simulink model "Indirect"  (R2015b)
settings: Solver=VariableStepAuto  StartTime=0.0  StopTime=7  RelTol=1e-3
values from neighbouring files (symbols this model uses):
  f = 50    [Indirect_init.m]
  L = XL/(2*2*pi*f)    (= 0.159154943092)    [Indirect_init.m]
  L_STATCOM = 44.56e-5    (= 0.0004456)    [Indirect_init.m]
  R_Statcom = 1e-1    (= 0.1)    [Indirect_init.m]
  Sbase = 1000e6/2    (= 500000000)    [Indirect_init.m]
  Ts = 10e-6    (= 1e-05)    [Indirect_init.m]
  Tsample = 200e-6    (= 0.0002)    [Indirect_init.m]
  Vr = 220e3    (= 220000)    [Indirect_init.m]
  Vs = 220e3    (= 220000)    [Indirect_init.m]
libraries: powerlib x27, powerlib_meascontrol x16, simulink x2
settings Model: Creator=Sourabh Suri  LastModifiedBy=Sourabh Suri

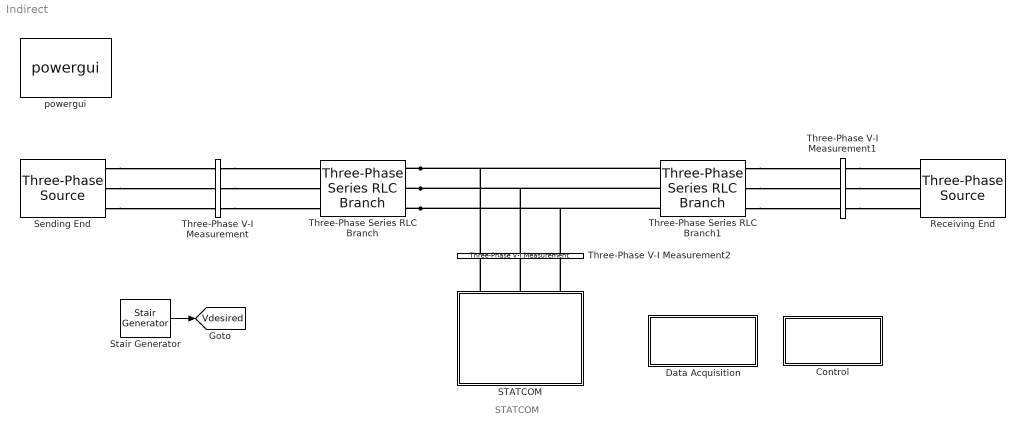
== system Indirect ==
  note: STATCOM
  Control : Subsystem
  Data Acquisition : Subsystem
  Receiving End : powerlib/Electrical Sources/Three-Phase Source  InternalConnection=Yg  VoltagePhases=off  Voltage=Vr  PhaseAngle=dr  Voltage_phases=[25e3 25e3 25e3]/sqrt(3)  PhaseAngles_phases=[0 -120 +120]  Frequency=f  NonIdealSource=off  SpecifyImpedance=off  Resistance=0.8929  Inductance=16.58e-3  ShortCircuitLevel=100e6  BaseVoltage=25e3  XRratio=7  BusType=swing  Pref=10e3  Qref=0  Prefabc=[10e3, 10e3, 10e3]  Qrefabc=[0, 0, 0]  Qmin=-inf  Qmax=inf
  STATCOM : Subsystem
  Sending End : powerlib/Electrical Sources/Three-Phase Source  InternalConnection=Yg  VoltagePhases=off  Voltage=Vs  PhaseAngle=ds  Voltage_phases=[25e3 25e3 25e3]/sqrt(3)  PhaseAngles_phases=[0 -120 +120]  Frequency=f  NonIdealSource=off  SpecifyImpedance=off  Resistance=0  Inductance=0  ShortCircuitLevel=100e6  BaseVoltage=0  XRratio=7  BusType=swing  Pref=10e3  Qref=0  Prefabc=[10e3, 10e3, 10e3]  Qrefabc=[0, 0, 0]  Qmin=-inf  Qmax=inf
  Stair Generator : powerlib_meascontrol/Pulse & Signal Generators/Stair Generator  t=[0:.5:.5*12]  e=[.07:.005:.13]  Ts=Ts
  Three-Phase Series RLC Branch : powerlib/Elements/Three-Phase Series RLC Branch  LConnTagsString=A|B|C  RConnTagsString=A|B|C  BranchType=L  Resistance=1  Inductance=L  Capacitance=1e-6  Measurements=None
  Three-Phase Series RLC Branch1 : powerlib/Elements/Three-Phase Series RLC Branch  LConnTagsString=A|B|C  RConnTagsString=A|B|C  BranchType=L  Resistance=1  Inductance=L  Capacitance=1e-6  Measurements=None
  Three-Phase V-I Measurement : powerlib/Measurements/Three-Phase V-I Measurement  VoltageMeasurement=phase-to-phase  SetLabelV=on  LabelV=Vsabc  Vpu=off  VpuLL=on  CurrentMeasurement=yes  SetLabelI=on  LabelI=Isabc  Ipu=on  Pbase=Sbase  Vbase=Vn  OutputType=Complex  PhasorSimulation=off  PSBequivalent=0
  Three-Phase V-I Measurement1 : powerlib/Measurements/Three-Phase V-I Measurement  VoltageMeasurement=phase-to-phase  SetLabelV=on  LabelV=Vrabc  Vpu=off  VpuLL=on  CurrentMeasurement=yes  SetLabelI=on  LabelI=Irabc  Ipu=on  Pbase=Sbase  Vbase=Vn  OutputType=Complex  PhasorSimulation=off  PSBequivalent=0
  Three-Phase V-I Measurement2 : powerlib/Measurements/Three-Phase V-I Measurement  VoltageMeasurement=phase-to-phase  SetLabelV=on  LabelV=Vmabc  Vpu=off  VpuLL=on  CurrentMeasurement=yes  SetLabelI=on  LabelI=Imabc  Ipu=on  Pbase=Sbase  Vbase=Vn  OutputType=Complex  PhasorSimulation=off  PSBequivalent=0
  powergui : powerlib/powergui  Priority=1  SimulationMode=Discrete  SolverType=Tustin/Backward Euler (TBE)  SampleTime=Ts  frequency=60  SPID=on  DisableSnubberDevices=on  DisableRonSwitches=on  DisableVfSwitches=on  SwTol=0  DisplayEquations=off  Interpol=off  ExternalGateDelay=off  methode=off  Ts=10  FunctionMessages=off  echomessages=off  HookPort=off  EnableUseOfTLC=off  x0status=blocks  frequencyindice=50  Pbase=100e6  ErrMax=1e-4  Iterations=50  UnitsV=kV  UnitsW=MW  buscounter=0  RestoreLinks=warning  ResistiveCurrentMeasurement=off  Frange=[0:2:500]  Ylog=off  Xlog=on  ShowGrid=off  save=off  variable=ZData  structure=0  ZoomFFT=off  StartTime=0.0  cycles=1  DisplayStyle=1  fundamental=60  FreqAxis=off  MaxFrequency=1000  frequencyindicesteady=1  RmsSteady=1  display=off
  tag scope: Vdesired=global
  wires:
  Stair Generator/1 -> [Vdesired]
  connections:
  Three-Phase Series RLC Branch/RConn1 -- Three-Phase Series RLC Branch1/RConn1 -- Three-Phase V-I Measurement2/RConn1
  Three-Phase Series RLC Branch/RConn2 -- Three-Phase Series RLC Branch1/RConn2 -- Three-Phase V-I Measurement2/RConn2
  Three-Phase Series RLC Branch/RConn3 -- Three-Phase Series RLC Branch1/RConn3 -- Three-Phase V-I Measurement2/RConn3
  Sending End/RConn1 -- Three-Phase V-I Measurement/LConn1
  Sending End/RConn2 -- Three-Phase V-I Measurement/LConn2
  Three-Phase V-I Measurement1/LConn2 -- Receiving End/RConn2
  Three-Phase Series RLC Branch1/LConn2 -- Three-Phase V-I Measurement1/RConn2
  Three-Phase V-I Measurement1/LConn1 -- Receiving End/RConn1
  Three-Phase Series RLC Branch1/LConn1 -- Three-Phase V-I Measurement1/RConn1
  Three-Phase V-I Measurement/RConn2 -- Three-Phase Series RLC Branch/LConn2
  Sending End/RConn3 -- Three-Phase V-I Measurement/LConn3
  Three-Phase V-I Measurement/RConn3 -- Three-Phase Series RLC Branch/LConn3
  Three-Phase Series RLC Branch1/LConn3 -- Three-Phase V-I Measurement1/RConn3
  Three-Phase V-I Measurement/RConn1 -- Three-Phase Series RLC Branch/LConn1
  Three-Phase V-I Measurement1/LConn3 -- Receiving End/RConn3
  STATCOM/LConn1 -- Three-Phase V-I Measurement2/LConn1
  STATCOM/LConn2 -- Three-Phase V-I Measurement2/LConn2
  STATCOM/LConn3 -- Three-Phase V-I Measurement2/LConn3

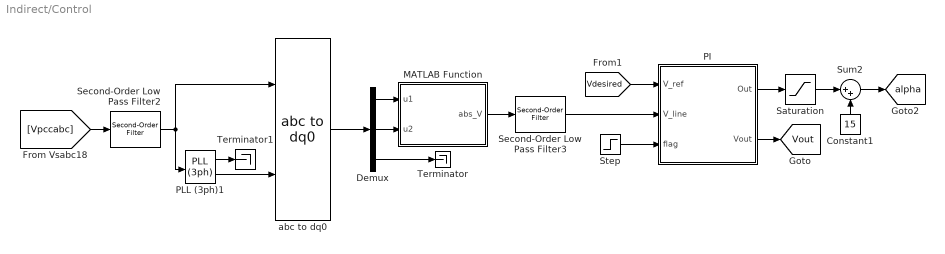
== system Indirect/Control ==
  Constant1 : Constant  Value=15
  Demux : Demux  Outputs=3
  MATLAB Function : MATLAB Function  TreatAsAtomicUnit=on
  PI : MATLAB Function  TreatAsAtomicUnit=on
  PLL (3ph)1 : powerlib_meascontrol/PLL/PLL (3ph)  Fmin=45  Par_Init=[3.7 50.1]  ParK=[60 1400 0]  TcD=1.6e-4  MaxRateChangeFreq=10  FilterCutOffFreq=25  Ts=Ts  AGC=on
  Saturation : Saturate  UpperLimit=45  LowerLimit=-15
  Second-Order Low Pass Filter2 : powerlib_meascontrol/Filters/Second-Order Filter  FilterType=Bandpass  Fo=50  Zeta=0.707  Ts=Ts  Initialize=off  Vac_Init="[0,  0,  60]"  Vdc_Init=0  PlotResponse=off  FreqRange=[0, 500, 1]
      settings: AttributesFormatString=f0: %<Fo>
  Second-Order Low Pass Filter3 : powerlib_meascontrol/Filters/Second-Order Filter  FilterType=Lowpass  Fo=25  Zeta=0.707  Ts=Ts  Initialize=off  Vac_Init="[0,  0,  60]"  Vdc_Init=0  PlotResponse=off  FreqRange=[0, 50, 1]
      settings: AttributesFormatString=f0: %<Fo>
  Step : Step  Time=1.01/f  SampleTime=0
  Sum2 : Sum  Inputs=|++  SaturateOnIntegerOverflow=on  InputSameDT=on  OutDataTypeStr=Inherit: Same as first input
  Terminator : Terminator
  Terminator1 : Terminator
  abc to dq0 : powerlib_meascontrol/Transformations/abc to dq0  Alignment=90 degrees behind phase A axis
  tag scope: Vout=global, alpha=global
  wires:
  [Vdesired] -> PI/1(V_ref)
  PI/1(Out) -> Saturation/1
  Saturation/1 -> Sum2/1
  Sum2/1 -> [alpha]
  Constant1/1 -> Sum2/2
  Step/1 -> PI/3(flag)
  PLL (3ph)1/2 -> abc to dq0/2
  [Vpccabc] -> Second-Order Low Pass Filter2/1
  abc to dq0/1 -> Demux/1
  Demux/1 -> MATLAB Function/1(u1)
  Demux/2 -> MATLAB Function/2(u2)
  Demux/3 -> Terminator/1
  Second-Order Low Pass Filter2/1 -> abc to dq0/1, PLL (3ph)1/1
  MATLAB Function/1(abs_V) -> Second-Order Low Pass Filter3/1
  Second-Order Low Pass Filter3/1 -> PI/2(V_line)
  PLL (3ph)1/1 -> Terminator1/1
  PI/2(Vout) -> [Vout]

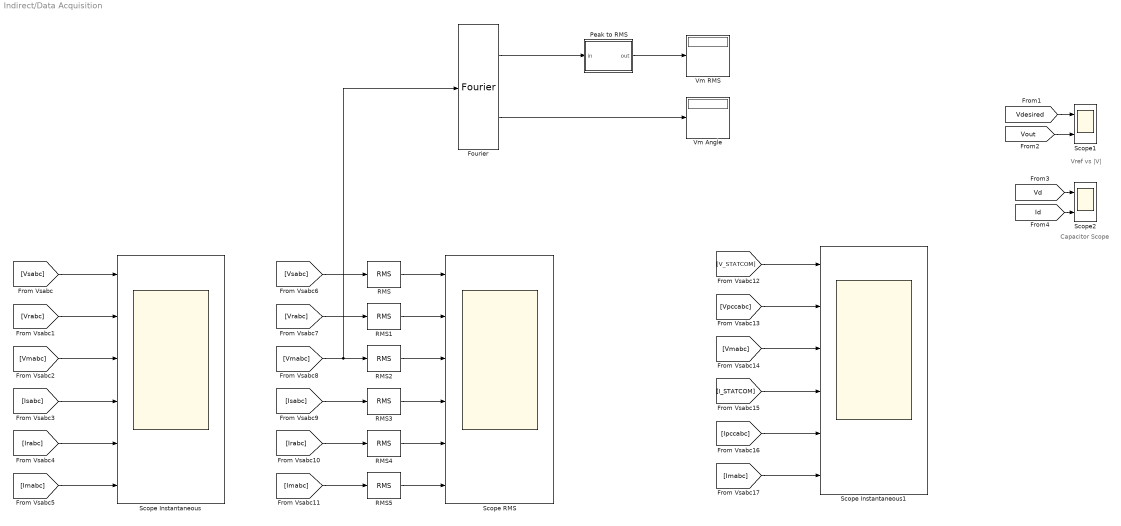
== system Indirect/Data Acquisition ==
  note: Vref vs |V|
  note: Capacitor Scope
  Fourier : powerlib_meascontrol/Measurements/Fourier  Freq=f  n=1  InInit=[0, 0]  Ts=0
  Peak to RMS : MATLAB Function  TreatAsAtomicUnit=on
  RMS{,1..5} (6 alike) : powerlib_meascontrol/Measurements/RMS  TrueRMS=off  Freq=f  RMSInit=0  Ts=0
  Scope Instantaneous : Scope  NumInputPorts=6
  Scope Instantaneous1 : Scope  NumInputPorts=6
  Scope RMS : Scope  NumInputPorts=6
  Scope1 : Scope  NumInputPorts=2
  Scope2 : Scope  NumInputPorts=2
  Vm Angle : Display
      settings: Decimation=3
  Vm RMS : Display
      settings: Decimation=3
  wires:
  [Vsabc] -> Scope Instantaneous/1
  [Vrabc] -> Scope Instantaneous/2
  [Irabc] -> Scope Instantaneous/5
  [Imabc] -> Scope Instantaneous/6
  [Vmabc] -> Scope Instantaneous/3
  [Isabc] -> Scope Instantaneous/4
  RMS/1 -> Scope RMS/1
  [Vrabc] -> RMS1/1
  RMS1/1 -> Scope RMS/2
  [Vmabc] -> Fourier/1, RMS2/1
  [Isabc] -> RMS3/1
  RMS3/1 -> Scope RMS/4
  [Irabc] -> RMS4/1
  RMS4/1 -> Scope RMS/5
  [Imabc] -> RMS5/1
  RMS5/1 -> Scope RMS/6
  RMS2/1 -> Scope RMS/3
  Fourier/2 -> Vm Angle/1
  [Vsabc] -> RMS/1
  Peak to RMS/1(out) -> Vm RMS/1
  Fourier/1 -> Peak to RMS/1(in)
  [Vdesired] -> Scope1/1
  [Vout] -> Scope1/2
  [Vd] -> Scope2/1
  [Id] -> Scope2/2
  [V_STATCOM] -> Scope Instantaneous1/1
  [Vpccabc] -> Scope Instantaneous1/2
  [Ipccabc] -> Scope Instantaneous1/5
  [Imabc] -> Scope Instantaneous1/6
  [Vmabc] -> Scope Instantaneous1/3
  [I_STATCOM] -> Scope Instantaneous1/4
  ? -> ?

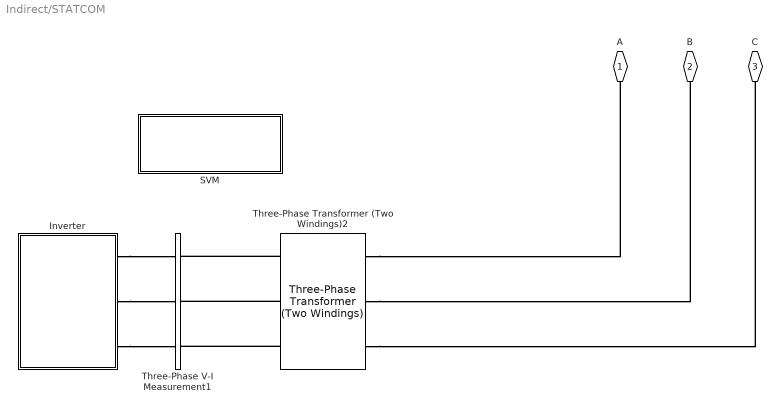
== system Indirect/STATCOM ==
  Inverter : Subsystem
  SVM : Subsystem
  Three-Phase Transformer (Two Windings)2 : powerlib/Elements/Three-Phase Transformer (Two Windings)  Winding1Connection=Y  Winding2Connection=Y  CoreType=Three-limb core (core-type)  SetSaturation=off  Hysteresis=off  DataFile='hysteresis'  SetInitialFlux=off  Measurements=None  UNITS=SI  NominalPower=[ Sbase*1000 , 50 ]  Winding1=[22e+04 1e-9 0 ]  Winding2=[22e+03 1e-9 0]  Rm=inf  Lm=inf  L0=0.5  Saturation=[0 0;4.3111 686.13;1796.3 869.1]  InitialFluxes=[457.42 -457.42 400.24]  MoreParameters=off  BreakLoop=off  DataType=on  TransfoNumber=1
  Three-Phase V-I Measurement1 : powerlib/Measurements/Three-Phase V-I Measurement  VoltageMeasurement=phase-to-phase  SetLabelV=on  LabelV=Vpccabc  Vpu=off  VpuLL=on  CurrentMeasurement=yes  SetLabelI=on  LabelI=Ipccabc  Ipu=on  Pbase=Sbase  Vbase=Vn  OutputType=Complex  PhasorSimulation=off  PSBequivalent=0
  A : PMIOPort  Port=1  Side=Left
  B : PMIOPort  Port=2  Side=Left
  C : PMIOPort  Port=3  Side=Left
  connections:
  Three-Phase Transformer (Two Windings)2/LConn1 -- A/RConn1
  Three-Phase Transformer (Two Windings)2/LConn2 -- B/RConn1
  Three-Phase Transformer (Two Windings)2/LConn3 -- C/RConn1
  Three-Phase Transformer (Two Windings)2/RConn1 -- Three-Phase V-I Measurement1/RConn1
  Three-Phase Transformer (Two Windings)2/RConn2 -- Three-Phase V-I Measurement1/RConn2
  Three-Phase Transformer (Two Windings)2/RConn3 -- Three-Phase V-I Measurement1/RConn3
  Inverter/LConn1 -- Three-Phase V-I Measurement1/LConn1
  Inverter/LConn2 -- Three-Phase V-I Measurement1/LConn2
  Inverter/LConn3 -- Three-Phase V-I Measurement1/LConn3

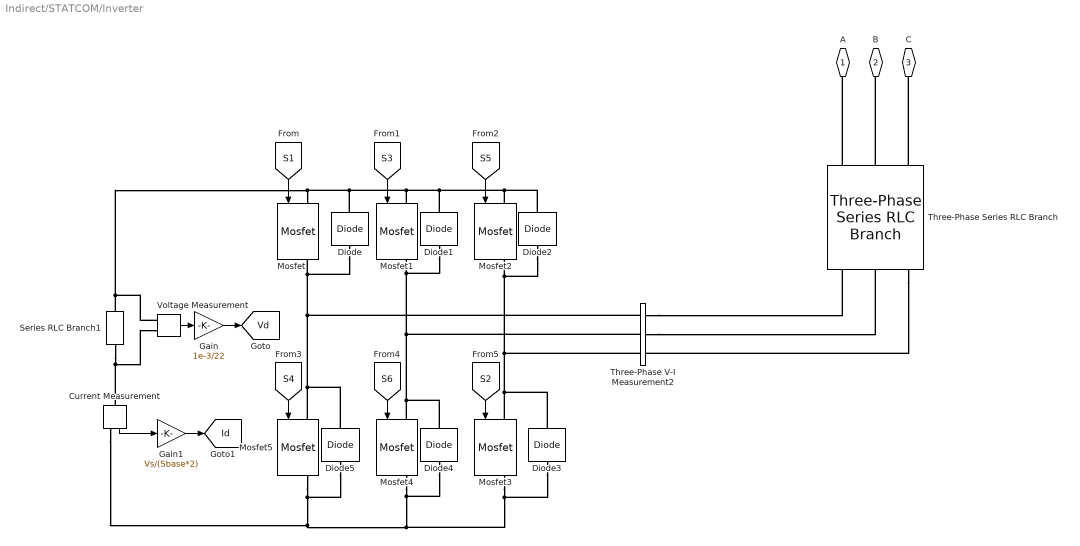
== system Indirect/STATCOM/Inverter ==
  Current Measurement : powerlib/Measurements/Current Measurement  PhasorSimulation=off  OutputType=Complex  PSBequivalent=0
  Diode{,1..5} (6 alike) : powerlib/Power Electronics/Diode  Ron=0.001  Lon=0  Vf=0.8  IC=0  UseSnubber=off  Rs=inf  Cs=250e-9  Measurements=off
  Gain : Gain  Gain=1e-3/22
  Gain1 : Gain  Gain=Vs/(Sbase*2)
  Mosfet{,1..5} (6 alike) : powerlib/Power Electronics/Mosfet  Ron=0.1  Lon=0  Rd=0.01  Vfd=0  IC=0  Rs=1e5  Cs=inf  Measurements=on
  Series RLC Branch1 : powerlib/Elements/Series RLC Branch  LConnTagsString=__new0  RConnTagsString=__new0  BranchType=C  Resistance=100  Inductance=1e-15  SetiL0=off  InitialCurrent=0  Capacitance=20e-4  Setx0=on  InitialVoltage=22e3/.45  Measurements=None
  Three-Phase Series RLC Branch : powerlib/Elements/Three-Phase Series RLC Branch  LConnTagsString=A|B|C  RConnTagsString=A|B|C  BranchType=RL  Resistance=R_Statcom  Inductance=L_STATCOM  Capacitance=1e-6  Measurements=None
  Three-Phase V-I Measurement2 : powerlib/Measurements/Three-Phase V-I Measurement  VoltageMeasurement=phase-to-phase  SetLabelV=on  LabelV=V_STATCOM  Vpu=off  VpuLL=on  CurrentMeasurement=yes  SetLabelI=on  LabelI=I_STATCOM  Ipu=on  Pbase=Sbase  Vbase=Vn  OutputType=Complex  PhasorSimulation=off  PSBequivalent=0
  Voltage Measurement : powerlib/Measurements/Voltage Measurement  PhasorSimulation=off  OutputType=Complex  PSBequivalent=0
  A : PMIOPort  Port=1  Side=Left
  B : PMIOPort  Port=2  Side=Left
  C : PMIOPort  Port=3  Side=Left
  tag scope: Id=global, Vd=global
  wires:
  [S2] -> Mosfet3/1
  [S4] -> Mosfet5/1
  [S1] -> Mosfet/1
  [S5] -> Mosfet2/1
  [S3] -> Mosfet1/1
  [S6] -> Mosfet4/1
  Voltage Measurement/1 -> Gain/1
  Gain/1 -> [Vd]
  Gain1/1 -> [Id]
  Current Measurement/1 -> Gain1/1
  connections:
  Series RLC Branch1/RConn1 -- Current Measurement/LConn1 -- Voltage Measurement/LConn2
  Voltage Measurement/LConn1 -- Series RLC Branch1/LConn1 -- Mosfet/LConn1 -- Diode2/RConn1 -- Mosfet2/LConn1 -- Diode1/RConn1 -- Mosfet1/LConn1 -- Diode/RConn1
  Mosfet/RConn1 -- Three-Phase V-I Measurement2/LConn1 -- Diode5/RConn1 -- Mosfet5/LConn1 -- Diode/LConn1
  Mosfet1/RConn1 -- Three-Phase V-I Measurement2/LConn2 -- Diode4/RConn1 -- Mosfet4/LConn1 -- Diode1/LConn1
  Mosfet2/RConn1 -- Three-Phase V-I Measurement2/LConn3 -- Diode3/RConn1 -- Mosfet3/LConn1 -- Diode2/LConn1
  Three-Phase Series RLC Branch/LConn2 -- B/RConn1
  Three-Phase Series RLC Branch/LConn3 -- C/RConn1
  Three-Phase Series RLC Branch/LConn1 -- A/RConn1
  Three-Phase V-I Measurement2/RConn1 -- Three-Phase Series RLC Branch/RConn1
  Three-Phase V-I Measurement2/RConn2 -- Three-Phase Series RLC Branch/RConn2
  Three-Phase Series RLC Branch/RConn3 -- Three-Phase V-I Measurement2/RConn3
  Diode3/LConn1 -- Current Measurement/RConn1 -- Diode5/LConn1 -- Mosfet5/RConn1 -- Diode4/LConn1 -- Mosfet4/RConn1 -- Mosfet3/RConn1

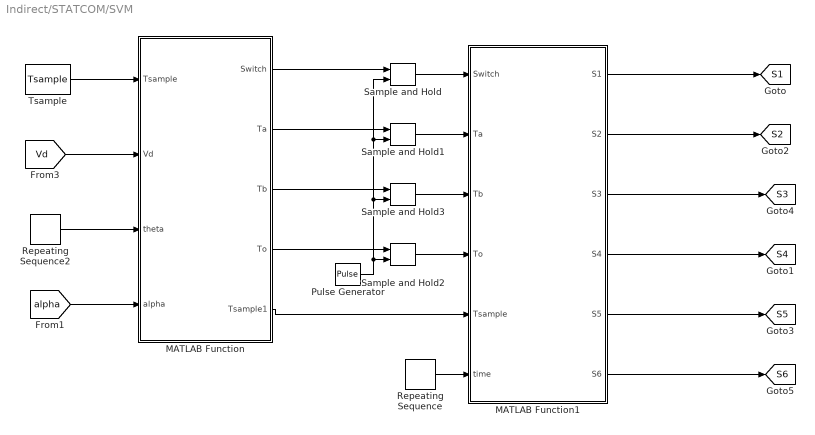
== system Indirect/STATCOM/SVM ==
  MATLAB Function : MATLAB Function  TreatAsAtomicUnit=on
  MATLAB Function1 : MATLAB Function  TreatAsAtomicUnit=on
  Pulse Generator : DiscretePulseGenerator  PulseType=Time based  Period=Tsample  PulseWidth=.1
  Repeating Sequence : simulink/Sources/Repeating Sequence  rep_seq_t=[0 Tsample ]  rep_seq_y=[0 Tsample]
  Repeating Sequence2 : simulink/Sources/Repeating Sequence  rep_seq_t=[0 1/f ]  rep_seq_y=[0 (2*pi)]
  Sample and Hold{,1..3} (4 alike) : powerlib_meascontrol/Additional Components/Sample and Hold  ic=0  Ts=Tsample
  Tsample : Constant  Value=Tsample
  tag scope: S1=global, S2=global, S3=global, S4=global, S5=global, S6=global
  wires:
  MATLAB Function/1(Switch) -> Sample and Hold/1
  Sample and Hold/1 -> MATLAB Function1/1(Switch)
  MATLAB Function/3(Tb) -> Sample and Hold3/1
  MATLAB Function1/1(S1) -> [S1]
  MATLAB Function1/5(S5) -> [S5]
  MATLAB Function1/3(S3) -> [S3]
  MATLAB Function1/4(S4) -> [S4]
  MATLAB Function1/2(S2) -> [S2]
  Sample and Hold1/1 -> MATLAB Function1/2(Ta)
  MATLAB Function/2(Ta) -> Sample and Hold1/1
  Sample and Hold2/1 -> MATLAB Function1/4(To)
  MATLAB Function/4(To) -> Sample and Hold2/1
  Pulse Generator/1 -> Sample and Hold/2, Sample and Hold1/2, Sample and Hold3/2, Sample and Hold2/2
  MATLAB Function1/6(S6) -> [S6]
  Tsample/1 -> MATLAB Function/1(Tsample)
  Repeating Sequence/1 -> MATLAB Function1/6(time)
  MATLAB Function/5(Tsample1) -> MATLAB Function1/5(Tsample)
  [Vd] -> MATLAB Function/2(Vd)
  Sample and Hold3/1 -> MATLAB Function1/3(Tb)
  Repeating Sequence2/1 -> MATLAB Function/3(theta)
  [alpha] -> MATLAB Function/4(alpha)

== matlab function Indirect/Control/MATLAB Function ==
  data: u1 input; u2 input; abs_V output
function abs_V = fcn(u1,u2)
%#codegen
abs_V= sqrt((u1*u1+u2*u2)/2);

== matlab function Indirect/Data Acquisition/Peak to RMS ==
  data: in input; out output
function out = fcn(in)
% converts peak values to RMS values

out = in/sqrt(2);

== matlab function Indirect/STATCOM/SVM/MATLAB Function ==
  data: Switch output; Ta output; Tb output; To output; Tsample1 output; Tsample input; Vd input; theta input; alpha input
function [Switch, Ta, Tb, To, Tsample1]= fcn(Tsample,Vd, theta, alpha)
%#codegen
Tsample1 = Tsample;
%magnitude = abs(Vref*cosine+Vref*1i* sine);
Vref= Vd*0.5;
Ta=0; Tb=0; To=0; %Tsample= 250e-6;

theta= theta+ 3*pi/2+(pi/90)+alpha*(pi/180);
Sector=1;
Switch = zeros(7,3);

if  theta>2*pi
    theta = -2*pi + theta;
end
if  theta<0
    theta = pi + theta;
end

if 0<theta && theta<=pi/3
    Sector= 1;
    
elseif pi/3<theta && theta<=2*pi/3
    Sector= 2;
    
elseif 2*pi/3<theta && theta<=pi
    Sector= 3;
    
elseif pi<theta && theta<=4*pi/3
    Sector= 4;
  
elseif 4*pi/3<theta && theta<=5*pi/3
    Sector= 5;
  
elseif 5*pi/3<theta && theta<=2*pi
    Sector= 6;

end
switch Sector
    case 1
     Ta = sqrt(3)* Tsample * Vref *sin((pi/3) - theta) / Vd;
     Tb = sqrt(3)* Tsample * Vref *sin(theta) / Vd;
     %To = Tsample - Ta - Tb;
     % Such that To/4, Ta/2, Tb/2, T0/2, Tb/2, Ta/2, To/2.
     % Here switching frequency will be sampling frequency
     % Van, Vbn, Vcn will be switched according to below sequence, 
     % 000, 100, 110, 111, 110, 100, 000.
     Switch = [0 0 0; 1 0 0; 1 1 0; 1 1 1; 1 1 0; 1 0 0; 0 0 0];
     
    case 2
     theta1 = theta - (pi/3);
     Ta = sqrt(3)* Tsample * Vref *sin((pi/3) - theta1) / Vd;
     Tb = sqrt(3)* Tsample * Vref *sin(theta1) / Vd;
     %To = Tsample - Ta - Tb;
     Switch = [0 0 0; 1 1 0; 0 1 0; 1 1 1; 0 1 0; 1 1 0; 0 0 0];
     
    case 3
     theta1 = theta - (2*pi/3);
     Ta = sqrt(3)* Tsample * Vref *sin((pi/3) - theta1) / Vd;
     Tb = sqrt(3)* Tsample * Vref *sin(theta1) / Vd;
     %To = Tsample - Ta - Tb;
     Switch = [0 0 0; 0 1 0; 0 1 1; 1 1 1; 0 1 1 ;0 1 0 ; 0 0 0];
     
    case 4
     theta1 = theta - (pi);
     Ta = sqrt(3)* Tsample * Vref *sin((pi/3) - theta1) / Vd;
     Tb = sqrt(3)* Tsample * Vref *sin(theta1) / Vd;
     %To = Tsample - Ta - Tb;
     Switch = [0 0 0;0 1 1; 0 0 1; 1 1 1; 0 0 1; 0 1 1; 0 0 0];
     
    case 5
     theta1 = theta - (4*pi/3);
     Ta = sqrt(3)* Tsample * Vref *sin((pi/3) - theta1) / Vd;
     Tb = sqrt(3)* Tsample * Vref *sin(theta1) / Vd;
     %To = Tsample - Ta - Tb;
     Switch = [0 0 0; 0 0 1; 1 0 1; 1 1 1; 1 0 1; 0 0 1; 0 0 0];
     
    case 6
     theta1 = theta - (5*pi/3);
     Ta = sqrt(3)* Tsample * Vref *sin((pi/3) - theta1) / Vd;
     Tb = sqrt(3)* Tsample * Vref *sin(theta1) / Vd;
     %To = Tsample - Ta - Tb;
     Switch = [0 0 0; 1 0 1; 1 0 0; 1 1 1; 1 0 0; 1 0 1; 0 0 0];
     
    otherwise
        Ta=0; Tb=0; To=0;
        
end
To = Tsample - Ta - Tb;
theta1= theta;

== matlab function Indirect/STATCOM/SVM/MATLAB Function1 ==
  data: Switch input; Ta input; Tb input; To input; Tsample input; S1 output; S2 output; S3 output; time input; S4 output; S5 output; S6 output
function [S1, S2, S3, S4, S5, S6] = fcn(Switch, Ta, Tb, To, Tsample,time)
%#codegen  To/4, Ta/2, Tb/2, T0/2, Tb/2, Ta/2, To/2.
%Tsample= 250e-6;
S1=0;
S2=0;
S3=0;
S4=0;
S5=0;
S6=0;
% if time1 > Tsample
%     time1 = 0;
% end
% time= time1+ t;
if (0< time) && (time<= To/4)
    S1 = Switch(1,1);
    S2 = Switch(1,2);
    S3 = Switch(1,3);
elseif (To/4 < time) && (time <= To/4 +  Ta/2)
    S1 = Switch(2,1);
    S2 = Switch(2,2);
    S3 = Switch(2,3);   
elseif (To/4 +  Ta/2 < time) && (time <  To/4 +  Ta/2 + Tb/2)
    S1 = Switch(3,1);
    S2 = Switch(3,2);
    S3 = Switch(3,3); 
elseif (To/4 +  Ta/2 + Tb/2  < time) && (time <  To/4 +  Ta/2 + Tb/2 + To/2)
    S1 = Switch(4,1);
    S2 = Switch(4,2);
    S3 = Switch(4,3); 
elseif (To/4 +  Ta/2 + Tb/2 + To/2 < time) && (time <  To/4 +  Ta/2 + Tb/2 + To/2 + Tb/2)
    S1 = Switch(5,1);
    S2 = Switch(5,2);
    S3 = Switch(5,3);
elseif (To/4 +  Ta/2 + Tb/2 + To/2 + Tb/2 < time) && (time < To/4 +  Ta/2 + Tb/2 + To/2 + Tb/2 + Ta/2)
    S1 = Switch(6,1);
    S2 = Switch(6,2);
    S3 = Switch(6,3);
elseif (To/4 +  Ta/2 + Tb/2 + To/2 + Tb/2 + Ta/2 < time) && (time <  To/4 +  Ta/2 + Tb/2 + To/2 + Tb/2 + Ta/2 + To/4)
    S1 = Switch(7,1);
    S2 = Switch(7,2);
    S3 = Switch(7,3);
end
S1=S1;
S4= 1-S1;
S5=S3;
S3=S2;
S2= 1-S5;
S6= 1-S3;

== matlab function Indirect/Control/PI ==
  data: V_ref input; Out output; V_line input; flag input; Vout output
function [Out,Vout] = fcn(V_ref,V_line,flag)
%V_line=V_line/3;
integrator=0;
differential=0;
Kp=400;
Ki=.22;
Kd=0;
%  Kp= 750;
% Ki= .022; %for L_STATCOM=1.3E3
% Kd= 0.1;
persistent error_old;
if(isempty(error_old))
    error_old=0;
end 
 
persistent Vi;
if(isempty(Vi))
    Vi=0;
end
persistent Vref;

if(isempty(Vref))
    Vref=0;
end

% if(Vref~=V_ref)
%     Vi=0; error=0;
%     integrator=0;
%     differential=0;
%     Vref=V_ref;
% end

error=V_ref-V_line;
if flag==1 
Vi=Vi+error;
differential= error - error_old;
integrator=Vi;
end 
 Out=-(Kp*error+Ki*Vi+Kd*differential);
 error_old = error;
Vout=V_line;
